simulink model "week1_7"  (R2020b)
settings: Solver=VariableStepAuto  StartTime=0.0  StopTime=10.0  RelTol=1e-3
settings Model: Creator=Lenovo  LastModifiedBy=Lenovo

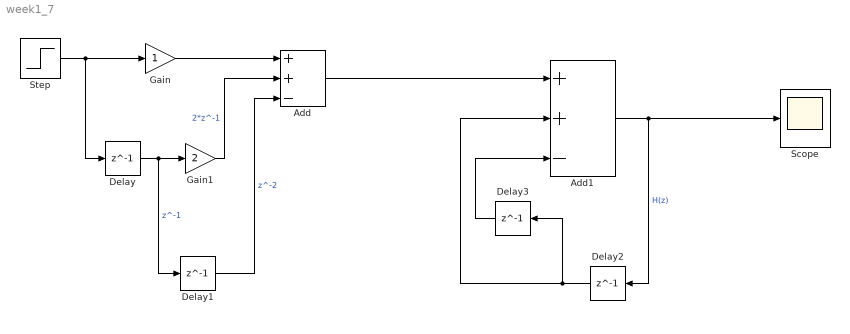
== system week1_7 ==
  Add : Sum  Inputs=++-
  Add1 : Sum  Inputs=++-
  Delay{,1..3} (4 alike) : Delay  DelayLength=1  InitialCondition=0
  Gain : Gain
  Gain1 : Gain  Gain=2
  Scope : Scope
  Step : Step  SampleTime=0
  wires:
  Step/1 -> Delay/1, Gain/1
  Delay/1 -> Delay1/1, Gain1/1  "z^-1"
  Gain1/1 -> Add/2  "2*z^-1"
  Gain/1 -> Add/1
  Delay1/1 -> Add/3  "z^-2"
  Add/1 -> Add1/1
  Delay2/1 -> Delay3/1, Add1/2
  Delay3/1 -> Add1/3
  Add1/1 -> Scope/1, Delay2/1  "H(z)"
